simulink model "DOO"  (R2020a)
settings: Solver=FixedStepAuto  StartTime=0.0  StopTime=10.0  FixedStep=1e-3  RelTol=1e-3  EnableMultiTasking=on
settings Model: ExtModeTrigDuration=5  Creator=Ethan  LastModifiedBy=Ethan
settings OptimizationCC: EnhancedBackFolding=on  PassReuseOutputArgsAs=Individual arguments  ZeroExternalMemoryAtStartup=off  ZeroInternalMemoryAtStartup=off  MaxStackSize=64  OptimizeBlockOrder=speed  DifferentSizesBufferReuse=on  OptimizationCustomize=off  EfficientTunableParamExpr=on
settings DebuggingCC: ParameterTunabilityLossMsg=error
settings HardwareCC: ProdBitPerPointer=32  ProdBitPerSizeT=32  ProdBitPerPtrDiffT=32  ProdLargestAtomicInteger=Long  ProdLargestAtomicFloat=Double  ProdWordSize=32  ProdHWDeviceType=ARM Compatible->ARM Cortex
settings SFSimCC: MATLABDynamicMemAlloc=off
settings RTWCC: SystemTargetFile=ert.tlc  HardwareBoard=NXP FRDM-K64F  TemplateMakefile=ert_default_tmf  Toolchain=GNU Tools for ARM Embedded Processors
settings CodeAppCC: ForceParamTrailComments=on  IgnoreCustomStorageClasses=off  OperatorAnnotations=on  SimulinkDataObjDesc=on  SFDataObjDesc=on  InsertBlockDesc=on

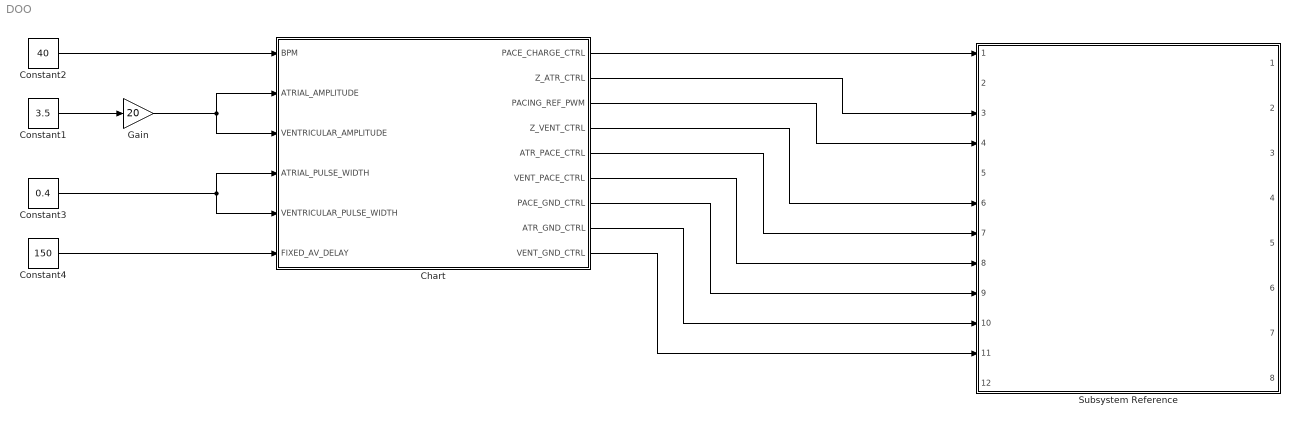
== system DOO ==
  Chart : Stateflow chart  TreatAsAtomicUnit=on
      settings: PortSchema="{\"entries\":[{\"content\":{\"sides\":[{\"content\":{\"connectorIds\":[\"In1\",\"In2\",\"In5\",\"In3\",\"In6\",\"In4\"]},\"type\":\"ConnectorPlacement.EquallySpacedRectSide\",\"uuid\":\"a22e05d8-b46e-41db-a99f-a3bab389e16c\"},{\"content\":{\"connectorIds\":[\"Out3\",\"Out8\",\"Out5\",\"Out9\",\"Out2\",\"Out7\",\"Out4\",\"Out1\",\"Out6\"],\"side\":\"RIGHT\"},\"type\":\"ConnectorPlacement.EquallySpacedRectSide\",\"uuid\":\"b830ec1d-656a-4b92-afcd-8fda6b31ad8a\"},{\"content\":{\"connectorIds\":[],\"side\":\"TOP\"},\"type\":\"ConnectorPlacement.EquallySpacedRectSide\",\"uuid\":\"956e5d71-b4a8-48ca-aae1-84adff4c1ec1\"}]},\"type\":\"ConnectorPlacement.EquallySpacedConnector\",\"uuid\":\"bd48be11-38ec-46b0-b71c-a53820608697\"}],\"packageUris\":[\"http://schema.mathworks.com/mf0/Connector/19700101\"],\"version\":\"1.0\"}"
  Constant1 : Constant  Value=3.5
  Constant2 : Constant  Value=40
  Constant3 : Constant  Value=0.4
  Constant4 : Constant  Value=150
  Gain : Gain  Gain=20
  Subsystem Reference : Subsystem  ReferencedSubsystem=k64f_subsystem
  wires:
  Constant2/1 -> Chart/1(BPM)
  Chart/1(ATR_GND_CTRL) -> Subsystem Reference/10
  Chart/6(VENT_GND_CTRL) -> Subsystem Reference/11
  Gain/1 -> Chart/5(VENTRICULAR_AMPLITUDE), Chart/2(ATRIAL_AMPLITUDE)
  Chart/4(PACE_GND_CTRL) -> Subsystem Reference/9
  Chart/9(Z_VENT_CTRL) -> Subsystem Reference/6
  Chart/3(PACE_CHARGE_CTRL) -> Subsystem Reference/1
  Chart/8(Z_ATR_CTRL) -> Subsystem Reference/3
  Chart/5(PACING_REF_PWM) -> Subsystem Reference/4
  Chart/7(VENT_PACE_CTRL) -> Subsystem Reference/8
  Constant3/1 -> Chart/3(ATRIAL_PULSE_WIDTH), Chart/6(VENTRICULAR_PULSE_WIDTH)
  Chart/2(ATR_PACE_CTRL) -> Subsystem Reference/7
  Constant1/1 -> Gain/1
  Constant4/1 -> Chart/4(FIXED_AV_DELAY)

== stateflow chart DOO/Chart ==
  state PULSE_ATR
    entry:
    PACE_CHARGE_CTRL = 0;
    PACE_GND_CTRL = 1;
    VENT_GND_CTRL = 0;
    VENT_PACE_CTRL = 0;
    Z_ATR_CTRL = 0;
    Z_VENT_CTRL = 0;
    ATR_GND_CTRL = 0;
    ATR_PACE_CTRL = 1;
  state CHARGE_ATR
    entry:
    ATR_PACE_CTRL = 0;
    VENT_PACE_CTRL = 0;
    PACING_REF_PWM = ATRIAL_AMPLITUDE;
    PACE_CHARGE_CTRL = 1;
  state DISCHARGE_ATR
    entry:
    PACE_GND_CTRL = 1;
    VENT_PACE_CTRL = 0;
    Z_ATR_CTRL = 0;
    Z_VENT_CTRL = 0;
    ATR_PACE_CTRL = 0;
    ATR_GND_CTRL = 0;
    VENT_GND_CTRL = 1;
  state PULSE_VENT
    entry:
    PACE_CHARGE_CTRL = 0;
    PACE_GND_CTRL = 1;
    VENT_GND_CTRL = 0;
    VENT_PACE_CTRL = 1;
    Z_ATR_CTRL = 0;
    Z_VENT_CTRL = 0;
    ATR_GND_CTRL = 0;
    ATR_PACE_CTRL = 0;
  state DISCHARGE_VENT
    entry:
    PACE_GND_CTRL = 1;
    VENT_PACE_CTRL = 0;
    Z_ATR_CTRL = 0;
    Z_VENT_CTRL = 0;
    ATR_PACE_CTRL = 0;
    ATR_GND_CTRL = 0;
    VENT_GND_CTRL = 1;
  state CHARGE_VENT
    entry:
    ATR_PACE_CTRL = 0;
    VENT_PACE_CTRL = 0;
    PACING_REF_PWM = VENTRICULAR_AMPLITUDE;
    PACE_CHARGE_CTRL = 1;
  (default) -> CHARGE_ATR
  CHARGE_ATR -> PULSE_ATR : after(60/BPM,sec)
  PULSE_ATR -> DISCHARGE_ATR : after(ATRIAL_PULSE_WIDTH, msec)
  DISCHARGE_VENT -> CHARGE_ATR
  DISCHARGE_ATR -> CHARGE_VENT
  PULSE_VENT -> DISCHARGE_VENT : after(VENTRICULAR_PULSE_WIDTH, msec)
  CHARGE_VENT -> PULSE_VENT : after(FIXED_AV_DELAY+ATRIAL_PULSE_WIDTH,msec)
  data: ATR_GND_CTRL output; ATR_PACE_CTRL output; PACE_CHARGE_CTRL output; PACE_GND_CTRL output; PACING_REF_PWM output; VENT_GND_CTRL output; VENT_PACE_CTRL output; Z_ATR_CTRL output; Z_VENT_CTRL output; BPM input; ATRIAL_AMPLITUDE input; ATRIAL_PULSE_WIDTH input; FIXED_AV_DELAY input; VENTRICULAR_AMPLITUDE input; VENTRICULAR_PULSE_WIDTH input
